simulink model "starshotsimv2"  (R2017a)
settings: Solver=VariableStepAuto  StartTime=0.0  StopTime=600  RelTol=1e-3
values from neighbouring files (symbols this model uses):
  B0 = 3.12e-5    (= 3.12e-05)    [starshot_DC_KD_setupv2.m]    (also in starshot_IC_initv2.m)
  G = 6.67e-11    [starshot_DC_KD_setupv2.m]    (also in starshot_IC_initv2.m)
  M_Earth = 5.972e24    (= 5.972e+24)    [starshot_DC_KD_setupv2.m]    (also in starshot_IC_initv2.m)
  mu_0 = 4*pi*(10^-7)    (= 1.25663706144e-06)    [starshot_DC_KD_setupv2.m]    (also in starshot_IC_initv2.m)
  n = 1000    [starshot_DC_KD_setupv2.m]    (also in starshot_IC_initv2.m = 500)
  omegacmd = [starshot.cmd.p,starshot.cmd.q,starshot.cmd.r]'    [starshot_IC_initv2.m]
  q0 = [qmatlab(2:4),qmatlab(1)]'    [starshot_DC_KD_setupv2.m]    (also in starshot_IC_initv2.m)
  R_Earth = 6.378e6    (= 6378000)    [starshot_DC_KD_setupv2.m]    (also in starshot_IC_initv2.m)
undefined symbols (not defined in the file or in its folder): qcmd, starshot
libraries: vrlib x2
settings Model: Creator=armen  LastModifiedBy=armen

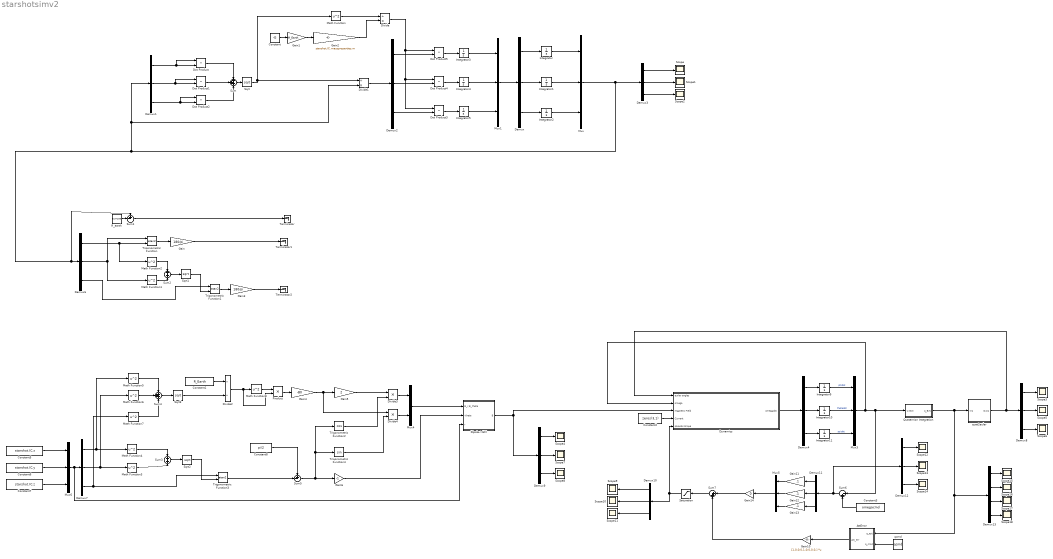
== system starshotsimv2 ==
  AttError : Subsystem
  Constant : Constant  Value=-G
  Constant1 : Constant  Value=R_Earth
  Constant2 : Constant  Value=zeros(3,1)
  Constant3 : Constant  Value=omegacmd
  Constant5 : Constant  Value=starshot.IC.x
  Constant6 : Constant  Value=starshot.IC.y
  Constant7 : Constant  Value=starshot.IC.z
  Constant8 : Constant  Value=pi/2
  Demux{,1..4,6..12} (12 alike) : Demux  Outputs=3
  Demux13 : Demux
  Dipole->ECI : Subsystem
  Divide : Product  Inputs=/*
  Divide1 : Product  Inputs=/*
  Divide2 : Product  Inputs=*/
  Divide3 : Product  Inputs=**
  Divide4 : Product  Inputs=**
  Dot Product{,1..5} (6 alike) : DotProduct  InputSameDT=on  OutDataTypeStr=Inherit: Inherit via internal rule
  Dynamics : Subsystem
  Gain : Gain  Gain=180/pi
  Gain1 : Gain  Gain=M_Earth
  Gain10 : Gain  Gain=[1,0,0;0,1,0;0,0,0,]  Multiplication=Matrix(K*u)
  Gain11 : Gain  Gain=.1
  Gain12 : Gain  Gain=.1
  Gain13 : Gain  Gain=.1
  Gain14 : Gain  Gain=0
  Gain2 : Gain  Gain=starshot.IC.massproperties.m
  Gain3 : Gain  Gain=180/pi
  Gain4 : Gain  Gain=-B0
  Gain5 : Gain  Gain=2
  Gain6 : Gain  Gain=-1
  Integrator : Integrator  InitialCondition=starshot.IC.x
  Integrator1 : Integrator  InitialCondition=starshot.IC.y
  Integrator10 : Integrator  InitialCondition=starshot.IC.thetadot
  Integrator11 : Integrator  InitialCondition=starshot.IC.psidot
  Integrator2 : Integrator  InitialCondition=starshot.IC.z
  Integrator3 : Integrator  InitialCondition=starshot.IC.xdot
  Integrator4 : Integrator  InitialCondition=starshot.IC.ydot
  Integrator5 : Integrator  InitialCondition=starshot.IC.zdot
  Integrator9 : Integrator  InitialCondition=starshot.IC.phidot
  Math Function{,1..8} (9 alike) : Math  Operator=square  SaturateOnIntegerOverflow=on
  Mux{,1,3,5..6} (5 alike) : Mux  Inputs=3
  Mux4 : Mux  Inputs=2
  Product : Product
  Quaternion Integration : Subsystem
  R_earth : Constant  Value=6.371e6
  Saturation : Saturate  UpperLimit=1e-4  LowerLimit=-1e-4
  Scope{,1..18} (19 alike) : Scope
  Sqrt{,1..3} (4 alike) : Sqrt  SaturateOnIntegerOverflow=on
  Sum : Sum  Inputs=+++
  Sum1 : Sum  Inputs=+-|
  Sum2 : Sum
  Sum3 : Sum
  Sum4 : Sum  Inputs=+++
  Sum5 : Sum  Inputs=+-|
  Sum6 : Sum  Inputs=|-+
  Sum7 : Sum  Inputs=|++
  Terminator : Terminator
  Terminator1 : Terminator
  Terminator2 : Terminator
  Trigonometric Function : Trigonometry  Operator=atan2
  Trigonometric Function1 : Trigonometry  Operator=atan2
  Trigonometric Function2 : Trigonometry  Operator=cos
  Trigonometric Function3 : Trigonometry  Operator=atan2
  Trigonometric Function4 : Trigonometry
  qcmd : Constant  Value=qcmd
  quat2euler : Subsystem
  wires:
  Integrator/1 -> Mux/1
  Integrator2/1 -> Mux/3
  Integrator1/1 -> Mux/2
  Demux/3 -> Integrator2/1
  Demux/2 -> Integrator1/1
  Demux/1 -> Integrator/1
  Mux1/1 -> Demux/1
  Integrator5/1 -> Mux1/3
  Integrator4/1 -> Mux1/2
  Integrator3/1 -> Mux1/1
  Demux1/1 -> Dot Product/1, Dot Product/2
  Demux1/2 -> Dot Product1/1, Dot Product1/2
  Demux1/3 -> Dot Product2/1, Dot Product2/2
  Dot Product1/1 -> Sum/2
  Dot Product2/1 -> Sum/3
  Dot Product/1 -> Sum/1
  Sum/1 -> Sqrt/1
  Constant/1 -> Gain1/1
  Sqrt/1 -> Math Function/1, Divide1/1
  Gain1/1 -> Gain2/1
  Gain2/1 -> Divide/2
  Math Function/1 -> Divide/1
  Divide/1 -> Dot Product3/1, Dot Product4/1, Dot Product5/1
  Demux2/3 -> Dot Product3/2
  Demux2/2 -> Dot Product4/2
  Demux2/1 -> Dot Product5/2
  Dot Product5/1 -> Integrator3/1
  Dot Product4/1 -> Integrator4/1
  Dot Product3/1 -> Integrator5/1
  Divide1/1 -> Demux2/1
  Demux3/1 -> Scope/1
  Demux3/2 -> Scope1/1
  Demux3/3 -> Scope2/1
  Integrator9/1 -> Mux3/1  "phidot"
  Integrator10/1 -> Mux3/2  "thetadot"
  Integrator11/1 -> Mux3/3  "psidot"
  Demux4/3 -> Integrator11/1
  Demux4/2 -> Integrator10/1
  Demux4/1 -> Integrator9/1
  Sum1/1 -> Terminator/1
  R_earth/1 -> Sum1/2
  Demux6/1 -> Math Function2/1, Trigonometric Function/2
  Demux6/2 -> Trigonometric Function/1, Math Function1/1
  Demux6/3 -> Trigonometric Function1/1
  Math Function2/1 -> Sum2/1
  Math Function1/1 -> Sum2/2
  Sum2/1 -> Sqrt1/1
  Sqrt1/1 -> Trigonometric Function1/2
  Trigonometric Function/1 -> Gain/1
  Trigonometric Function1/1 -> Gain3/1
  Gain/1 -> Terminator1/1
  Gain3/1 -> Terminator2/1
  Dynamics/1(omegadot) -> Demux4/1
  Sqrt2/1 -> Trigonometric Function3/2
  Sum3/1 -> Sqrt2/1
  Math Function3/1 -> Sum3/2
  Math Function4/1 -> Sum3/1
  Demux7/3 -> Math Function7/1, Trigonometric Function3/1
  Demux7/2 -> Math Function6/1, Math Function3/1
  Demux7/1 -> Math Function5/1, Math Function4/1
  Mux/1 -> Sum1/1, Demux6/1, Divide1/2, Demux1/1, Demux3/1
  Math Function6/1 -> Sum4/2
  Math Function5/1 -> Sum4/1
  Math Function7/1 -> Sum4/3
  Sum4/1 -> Sqrt3/1
  Sqrt3/1 -> Divide2/2
  Constant1/1 -> Divide2/1
  Divide2/1 -> Product/2, Math Function8/1
  Math Function8/1 -> Product/1
  Product/1 -> Gain4/1
  Gain4/1 -> Gain5/1, Divide4/1
  Gain5/1 -> Divide3/1
  Trigonometric Function2/1 -> Divide3/2
  Trigonometric Function4/1 -> Divide4/2
  Divide3/1 -> Mux4/1
  Divide4/1 -> Mux4/2
  Mux4/1 -> Dipole->ECI/1(B_r,B_theta)
  Gain6/1 -> Dipole->ECI/2(-theta)
  Demux9/3 -> Scope8/1
  Demux9/1 -> Scope4/1
  Demux9/2 -> Scope7/1
  Dipole->ECI/1(B) -> Demux9/1, Dynamics/3(Magnetic Field)
  Mux6/1 -> Dipole->ECI/3(r), Demux7/1
  Constant7/1 -> Mux6/3
  Constant6/1 -> Mux6/2
  Constant5/1 -> Mux6/1
  Demux8/2 -> Scope5/1
  Demux8/1 -> Scope3/1
  Demux8/3 -> Scope6/1
  Trigonometric Function3/1 -> Sum5/2
  Constant8/1 -> Sum5/1
  Sum5/1 -> Trigonometric Function2/1, Trigonometric Function4/1, Gain6/1
  quat2euler/1(Out1) -> Dynamics/1(eurler angles), Demux8/1
  AttError/1(att_err) -> Gain10/1
  qcmd/1 -> AttError/2(q_cmd)
  Constant2/1 -> Dynamics/4("Current ")
  Gain10/1 -> Sum7/2
  Demux10/1 -> Scope9/1
  Demux10/2 -> Scope10/1
  Demux10/3 -> Scope11/1
  Demux11/3 -> Gain13/1
  Gain13/1 -> Mux5/3
  Demux11/2 -> Gain12/1
  Gain12/1 -> Mux5/2
  Demux11/1 -> Gain11/1
  Gain11/1 -> Mux5/1
  Mux5/1 -> Gain14/1
  Sum6/1 -> Demux12/1, Demux11/1
  Constant3/1 -> Sum6/2
  Gain14/1 -> Sum7/1
  Sum7/1 -> Saturation/1
  Saturation/1 -> Demux10/1, Dynamics/5(pseudo-torque)
  Mux3/1 -> Dynamics/2(omega), Sum6/1, Quaternion Integration/1(w B/N)
  Demux12/3 -> Scope14/1
  Demux12/1 -> Scope12/1
  Demux12/2 -> Scope13/1
  Quaternion Integration/1(q_B/N) -> AttError/1(q_est), Demux13/1, quat2euler/1(In1)
  Demux13/1 -> Scope15/1
  Demux13/2 -> Scope16/1
  Demux13/3 -> Scope17/1
  Demux13/4 -> Scope18/1

== system starshotsimv2/AttError ==
  q_est : Inport  PortDimensions=4
  q_cmd : Inport  Port=2  PortDimensions=4
  Demux : Demux
  Gain : Gain  Gain=2  SaturateOnIntegerOverflow=on  OutDataTypeStr=Inherit: Same as input  ParamDataTypeStr=Inherit: Same as input
  Mux : Mux  Inputs=3
  Terminator : Terminator
  qconjMult : Subsystem
  att_err : Outport
  wires:
  Demux/4 -> Terminator/1
  Gain/1 -> att_err/1
  Mux/1 -> Gain/1
  Demux/3 -> Mux/3
  Demux/2 -> Mux/2
  Demux/1 -> Mux/1
  qconjMult/1(q_err) -> Demux/1
  q_est/1 -> qconjMult/2(q_est)
  q_cmd/1 -> qconjMult/1(q_cmd)

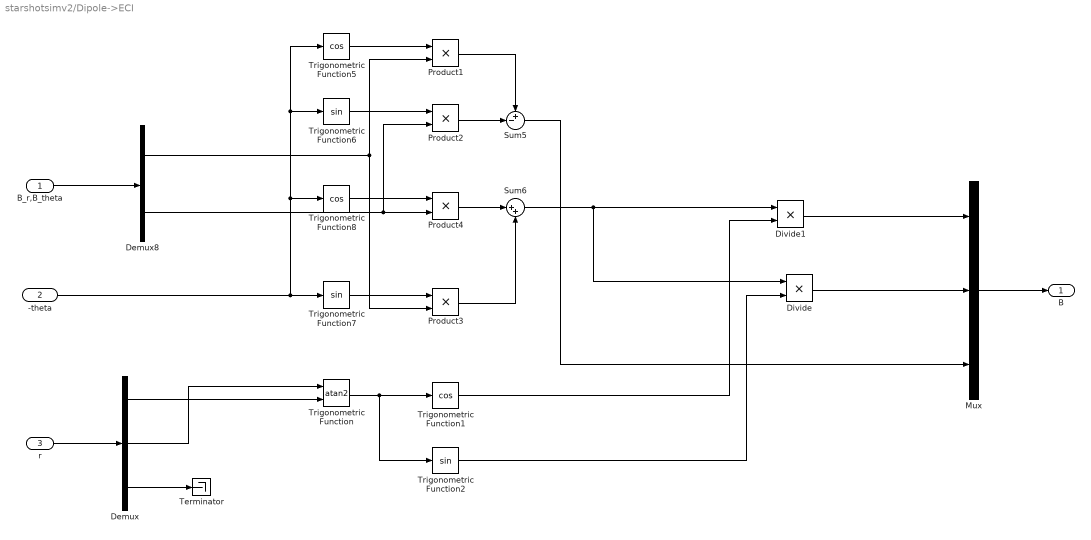
== system starshotsimv2/Dipole->ECI ==
  B_r,B_theta : Inport
  -theta : Inport  Port=2
  r : Inport  Port=3
  Demux : Demux  Outputs=3
  Demux8 : Demux  Outputs=2
  Divide : Product  Inputs=**
  Divide1 : Product  Inputs=**
  Mux : Mux  Inputs=3
  Product{1..4} (4 alike) : Product
  Sum5 : Sum  Inputs=+-|
  Sum6 : Sum  Inputs=|++
  Terminator : Terminator
  Trigonometric Function : Trigonometry  Operator=atan2
  Trigonometric Function1 : Trigonometry  Operator=cos
  Trigonometric Function2 : Trigonometry
  Trigonometric Function5 : Trigonometry  Operator=cos
  Trigonometric Function6 : Trigonometry
  Trigonometric Function7 : Trigonometry
  Trigonometric Function8 : Trigonometry  Operator=cos
  B : Outport
  wires:
  -theta/1 -> Trigonometric Function5/1, Trigonometric Function6/1, Trigonometric Function8/1, Trigonometric Function7/1
  Product4/1 -> Sum6/1
  Product3/1 -> Sum6/2
  Demux8/1 -> Product3/2, Product1/2
  Demux8/2 -> Product2/2, Product4/2
  Trigonometric Function5/1 -> Product1/1
  Product2/1 -> Sum5/2
  Trigonometric Function7/1 -> Product3/1
  B_r,B_theta/1 -> Demux8/1
  Sum5/1 -> Mux/3
  Trigonometric Function8/1 -> Product4/1
  Trigonometric Function6/1 -> Product2/1
  Sum6/1 -> Divide1/1, Divide/1
  Product1/1 -> Sum5/1
  r/1 -> Demux/1
  Demux/3 -> Terminator/1
  Demux/2 -> Trigonometric Function/1
  Demux/1 -> Trigonometric Function/2
  Trigonometric Function/1 -> Trigonometric Function1/1, Trigonometric Function2/1
  Trigonometric Function1/1 -> Divide1/2
  Trigonometric Function2/1 -> Divide/2
  Mux/1 -> B/1
  Divide1/1 -> Mux/1
  Divide/1 -> Mux/2

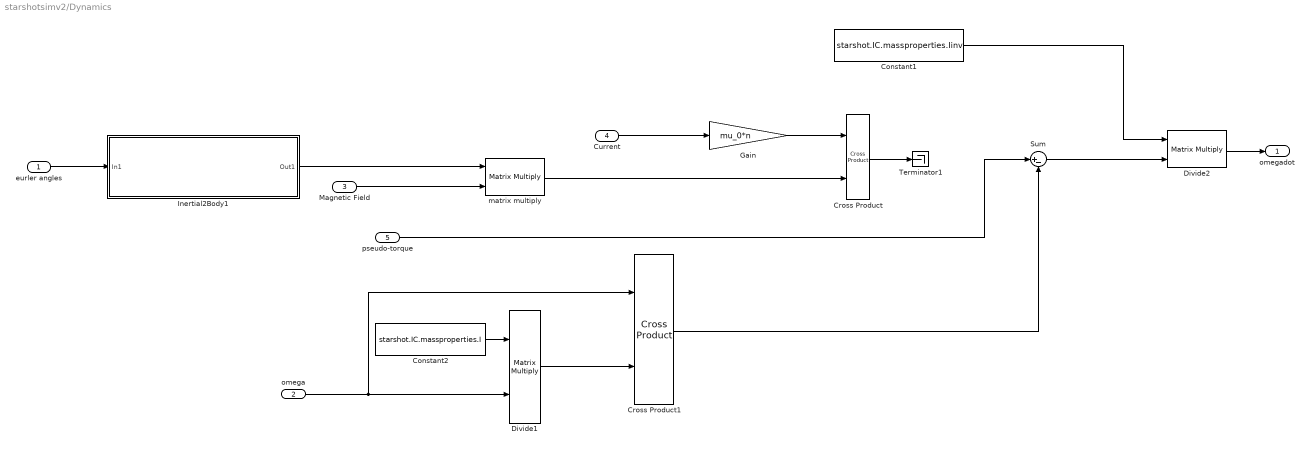
== system starshotsimv2/Dynamics ==
  eurler angles : Inport
  omega : Inport  Port=2
  Magnetic Field : Inport  Port=3
  "Current " : Inport  Port=4
  pseudo-torque : Inport  Port=5
  Constant1 : Constant  Value=starshot.IC.massproperties.Iinv  VectorParams1D=off
  Constant2 : Constant  Value=starshot.IC.massproperties.I  VectorParams1D=off
  Cross Product : vrlib/Utilities/Cross Product
      settings: SourceProductBaseCode=VR
  Cross Product1 : vrlib/Utilities/Cross Product
      settings: SourceProductBaseCode=VR
  Divide1 : Product  Inputs=**  Multiplication=Matrix(*)
  Divide2 : Product  Inputs=**  Multiplication=Matrix(*)
  Gain : Gain  Gain=mu_0*n
  Inertial2Body1 : Subsystem
  Sum : Sum  Inputs=|+-
  Terminator1 : Terminator
  "matrix multiply " : Product  Inputs=**  Multiplication=Matrix(*)
  omegadot : Outport
  wires:
  eurler angles/1 -> Inertial2Body1/1(In1)
  Inertial2Body1/1(Out1) -> "matrix multiply "/1
  omega/1 -> Divide1/2, Cross Product1/1
  Constant2/1 -> Divide1/1
  Magnetic Field/1 -> "matrix multiply "/2
  "Current "/1 -> Gain/1
  "matrix multiply "/1 -> Cross Product/2
  Gain/1 -> Cross Product/1
  Cross Product/1 -> Terminator1/1
  Divide1/1 -> Cross Product1/2
  Cross Product1/1 -> Sum/2
  Sum/1 -> Divide2/2
  Constant1/1 -> Divide2/1
  Divide2/1 -> omegadot/1
  pseudo-torque/1 -> Sum/1

== system starshotsimv2/Quaternion Integration ==
  w B/N : Inport
  Integrator1 : Integrator  InitialCondition=q0
  q_normalize : Subsystem
  qderiv : Subsystem
  q_B/N : Outport
  wires:
  w B/N/1 -> qderiv/1(w)
  q_normalize/1(q_out) -> qderiv/2(q), q_B/N/1
  Integrator1/1 -> q_normalize/1(q_in)
  qderiv/1(qd) -> Integrator1/1

== system starshotsimv2/quat2euler ==
  In1 : Inport
  Mux : Mux  Inputs=3
  Subsystem : Subsystem
  Subsystem1 : Subsystem
  q2phi : Subsystem
  Out1 : Outport
  wires:
  In1/1 -> Subsystem/1(q), Subsystem1/1(q), q2phi/1(q)
  Mux/1 -> Out1/1
  q2phi/1(phi) -> Mux/1
  Subsystem1/1(theta) -> Mux/2
  Subsystem/1(psi) -> Mux/3

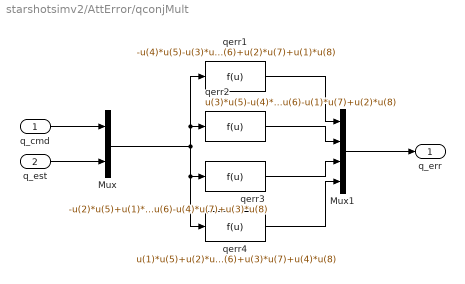
== system starshotsimv2/AttError/qconjMult ==
  q_cmd : Inport
  q_est : Inport  Port=2
  Mux : Mux  Inputs=2
  Mux1 : Mux
  qerr1 : Fcn  Expr=-u(4)*u(5)-u(3)*u(6)+u(2)*u(7)+u(1)*u(8)
  qerr2 : Fcn  Expr=u(3)*u(5)-u(4)*u(6)-u(1)*u(7)+u(2)*u(8)
  qerr3 : Fcn  Expr=-u(2)*u(5)+u(1)*u(6)-u(4)*u(7)+u(3)*u(8)
  qerr4 : Fcn  Expr=u(1)*u(5)+u(2)*u(6)+u(3)*u(7)+u(4)*u(8)
  q_err : Outport
  wires:
  Mux1/1 -> q_err/1
  qerr4/1 -> Mux1/4
  qerr3/1 -> Mux1/3
  qerr2/1 -> Mux1/2
  qerr1/1 -> Mux1/1
  Mux/1 -> qerr4/1, qerr3/1, qerr2/1, qerr1/1
  q_est/1 -> Mux/2
  q_cmd/1 -> Mux/1

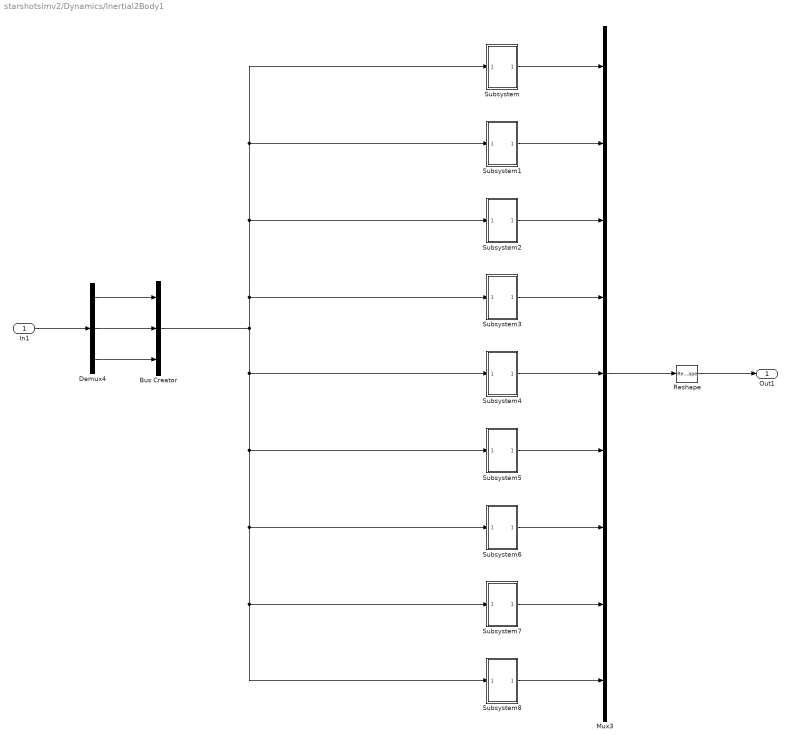
== system starshotsimv2/Dynamics/Inertial2Body1 ==
  In1 : Inport
  Bus Creator : BusCreator  Inputs=3
  Demux4 : Demux  Outputs=3
  Mux3 : Mux  Inputs=9
  Reshape : Reshape  OutputDimensionality=Customize  OutputDimensions=[3,3]
  Subsystem : Subsystem
  Subsystem1 : Subsystem
  Subsystem2 : Subsystem
  Subsystem3 : Subsystem
  Subsystem4 : Subsystem
  Subsystem5 : Subsystem
  Subsystem6 : Subsystem
  Subsystem7 : Subsystem
  Subsystem8 : Subsystem
  Out1 : Outport
  wires:
  Reshape/1 -> Out1/1
  Subsystem3/1(Out1) -> Mux3/4
  Subsystem4/1(Out1) -> Mux3/5
  Subsystem6/1(Out1) -> Mux3/7
  Subsystem2/1(Out1) -> Mux3/3
  Subsystem8/1(Out1) -> Mux3/9
  Subsystem7/1(Out1) -> Mux3/8
  Subsystem5/1(Out1) -> Mux3/6
  Subsystem1/1(Out1) -> Mux3/2
  Subsystem/1(Out1) -> Mux3/1
  Bus Creator/1 -> Subsystem4/1(In1), Subsystem5/1(In1), Subsystem8/1(In1), Subsystem7/1(In1), Subsystem6/1(In1), Subsystem3/1(In1), Subsystem1/1(In1), Subsystem/1(In1), Subsystem2/1(In1)
  Demux4/3 -> Bus Creator/3
  In1/1 -> Demux4/1
  Demux4/1 -> Bus Creator/1
  Demux4/2 -> Bus Creator/2
  Mux3/1 -> Reshape/1

== system starshotsimv2/Quaternion Integration/q_normalize ==
  q_in : Inport  PortDimensions=4
  Dot Product : DotProduct  InputSameDT=on  OutDataTypeStr=Inherit: Inherit via internal rule
  Math Function : Math  Operator=sqrt  SaturateOnIntegerOverflow=on
  Product : Product  Inputs=*/  SaturateOnIntegerOverflow=on  InputSameDT=on  OutDataTypeStr=Inherit: Same as first input
  q_out : Outport
  wires:
  Product/1 -> q_out/1
  Math Function/1 -> Product/2
  Dot Product/1 -> Math Function/1
  q_in/1 -> Dot Product/2, Dot Product/1, Product/1

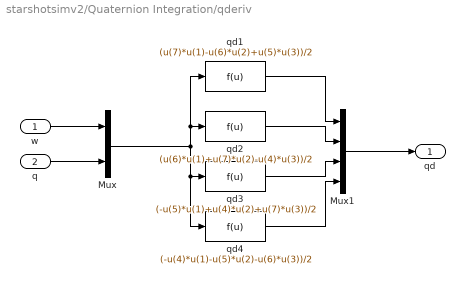
== system starshotsimv2/Quaternion Integration/qderiv ==
  w : Inport
  q : Inport  Port=2
  Mux : Mux  Inputs=2
  Mux1 : Mux
  qd1 : Fcn  Expr=(u(7)*u(1)-u(6)*u(2)+u(5)*u(3))/2
  qd2 : Fcn  Expr=(u(6)*u(1)+u(7)*u(2)-u(4)*u(3))/2
  qd3 : Fcn  Expr=(-u(5)*u(1)+u(4)*u(2)+u(7)*u(3))/2
  qd4 : Fcn  Expr=(-u(4)*u(1)-u(5)*u(2)-u(6)*u(3))/2
  qd : Outport
  wires:
  Mux1/1 -> qd/1
  qd4/1 -> Mux1/4
  qd3/1 -> Mux1/3
  qd2/1 -> Mux1/2
  qd1/1 -> Mux1/1
  Mux/1 -> qd4/1, qd3/1, qd2/1, qd1/1
  q/1 -> Mux/2
  w/1 -> Mux/1

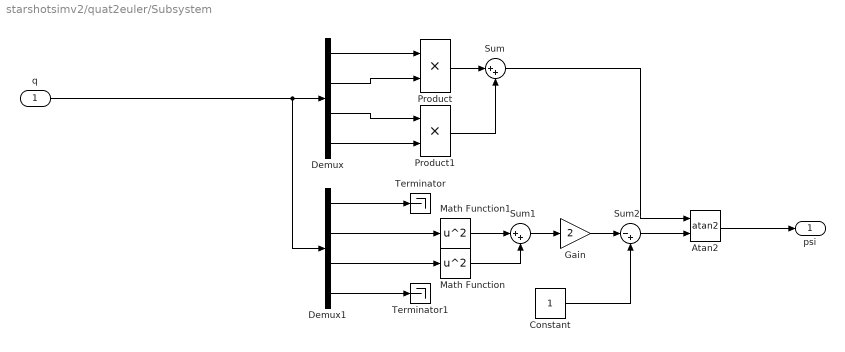
== system starshotsimv2/quat2euler/Subsystem ==
  q : Inport
  Atan2 : Trigonometry  Operator=atan2
  Constant : Constant
  Demux : Demux
  Demux1 : Demux
  Gain : Gain  Gain=2
  Math Function : Math  Operator=square  SaturateOnIntegerOverflow=on
  Math Function1 : Math  Operator=square  SaturateOnIntegerOverflow=on
  Product : Product
  Product1 : Product
  Sum : Sum  Inputs=|++
  Sum1 : Sum  Inputs=|++
  Sum2 : Sum  Inputs=|-+
  Terminator : Terminator
  Terminator1 : Terminator
  psi : Outport
  wires:
  Sum2/1 -> Atan2/2
  Math Function1/1 -> Sum1/1
  Demux/2 -> Product/2
  Demux/3 -> Product1/1
  Demux/4 -> Product1/2
  Product1/1 -> Sum/2
  Product/1 -> Sum/1
  Sum1/1 -> Gain/1
  Atan2/1 -> psi/1
  Sum/1 -> Atan2/1
  Demux1/2 -> Math Function1/1
  Demux1/4 -> Terminator1/1
  q/1 -> Demux1/1, Demux/1
  Demux1/3 -> Math Function/1
  Gain/1 -> Sum2/1
  Demux/1 -> Product/1
  Demux1/1 -> Terminator/1
  Constant/1 -> Sum2/2
  Math Function/1 -> Sum1/2

== system starshotsimv2/quat2euler/Subsystem1 ==
  q : Inport
  Demux : Demux
  Gain : Gain  Gain=2
  Product : Product
  Product1 : Product
  Sum : Sum  Inputs=-+|
  Trigonometric Function : Trigonometry  Operator=asin
  theta : Outport
  wires:
  Sum/1 -> Gain/1
  Trigonometric Function/1 -> theta/1
  Demux/2 -> Product/1
  Product1/1 -> Sum/1
  Gain/1 -> Trigonometric Function/1
  Demux/1 -> Product1/1
  Demux/4 -> Product/2
  Demux/3 -> Product1/2
  Product/1 -> Sum/2
  q/1 -> Demux/1

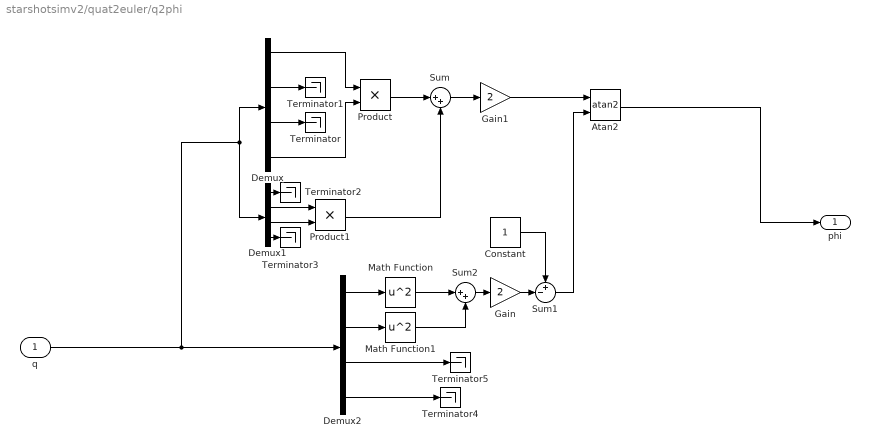
== system starshotsimv2/quat2euler/q2phi ==
  q : Inport
  Atan2 : Trigonometry  Operator=atan2
  Constant : Constant
  Demux : Demux
  Demux1 : Demux
  Demux2 : Demux
  Gain : Gain  Gain=2
  Gain1 : Gain  Gain=2
  Math Function : Math  Operator=square  SaturateOnIntegerOverflow=on
  Math Function1 : Math  Operator=square  SaturateOnIntegerOverflow=on
  Product : Product
  Product1 : Product
  Sum : Sum  Inputs=|++
  Sum1 : Sum  Inputs=+-|
  Sum2 : Sum  Inputs=|++
  Terminator{,1..5} (6 alike) : Terminator
  phi : Outport
  wires:
  Demux2/4 -> Terminator4/1
  Demux1/2 -> Product1/1
  Product/1 -> Sum/1
  Demux2/1 -> Math Function/1
  Atan2/1 -> phi/1
  Sum/1 -> Gain1/1
  Demux/3 -> Terminator/1
  Demux1/4 -> Terminator3/1
  Demux2/3 -> Terminator5/1
  Product1/1 -> Sum/2
  Demux/2 -> Terminator1/1
  Demux1/1 -> Terminator2/1
  Demux/4 -> Product/2
  Demux1/3 -> Product1/2
  Demux/1 -> Product/1
  Math Function1/1 -> Sum2/2
  Sum2/1 -> Gain/1
  Demux2/2 -> Math Function1/1
  Gain/1 -> Sum1/2
  Constant/1 -> Sum1/1
  Gain1/1 -> Atan2/1
  Sum1/1 -> Atan2/2
  q/1 -> Demux1/1, Demux/1, Demux2/1
  Math Function/1 -> Sum2/1

== system starshotsimv2/Dynamics/Inertial2Body1/Subsystem ==
  In1 : Inport
  Bus Selector : BusSelector  OutputSignals=signal1,signal3
  Product4 : Product
  Trigonometric Function : Trigonometry  Operator=cos
  Trigonometric Function1 : Trigonometry  Operator=cos
  Out1 : Outport
  wires:
  In1/1 -> Bus Selector/1
  Product4/1 -> Out1/1
  Trigonometric Function/1 -> Product4/1
  Trigonometric Function1/1 -> Product4/2
  Bus Selector/1 -> Trigonometric Function/1  "<signal1>"
  Bus Selector/2 -> Trigonometric Function1/1  "<signal3>"

== system starshotsimv2/Dynamics/Inertial2Body1/Subsystem1 ==
  In1 : Inport
  Bus Selector1 : BusSelector  OutputSignals=signal1,signal3
  Product5 : Product
  Trigonometric Function2 : Trigonometry  Operator=cos
  Trigonometric Function3 : Trigonometry
  Out1 : Outport
  wires:
  In1/1 -> Bus Selector1/1
  Product5/1 -> Out1/1
  Trigonometric Function2/1 -> Product5/1
  Bus Selector1/1 -> Trigonometric Function2/1  "<signal1>"
  Trigonometric Function3/1 -> Product5/2
  Bus Selector1/2 -> Trigonometric Function3/1  "<signal3>"

== system starshotsimv2/Dynamics/Inertial2Body1/Subsystem2 ==
  In1 : Inport
  Bus Selector2 : BusSelector  OutputSignals=signal3
  Gain : Gain  Gain=-1
  Trigonometric Function4 : Trigonometry
  Out1 : Outport
  wires:
  Gain/1 -> Out1/1
  In1/1 -> Bus Selector2/1
  Bus Selector2/1 -> Trigonometric Function4/1  "<signal3>"
  Trigonometric Function4/1 -> Gain/1

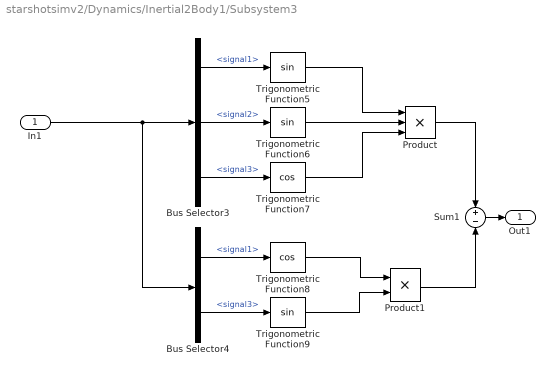
== system starshotsimv2/Dynamics/Inertial2Body1/Subsystem3 ==
  In1 : Inport
  Bus Selector3 : BusSelector  OutputSignals=signal1,signal2,signal3
  Bus Selector4 : BusSelector  OutputSignals=signal1,signal3
  Product : Product  Inputs=3
  Product1 : Product
  Sum1 : Sum  Inputs=+-
  Trigonometric Function5 : Trigonometry
  Trigonometric Function6 : Trigonometry
  Trigonometric Function7 : Trigonometry  Operator=cos
  Trigonometric Function8 : Trigonometry  Operator=cos
  Trigonometric Function9 : Trigonometry
  Out1 : Outport
  wires:
  Sum1/1 -> Out1/1
  In1/1 -> Bus Selector3/1, Bus Selector4/1
  Trigonometric Function7/1 -> Product/3
  Trigonometric Function9/1 -> Product1/2
  Product/1 -> Sum1/1
  Product1/1 -> Sum1/2
  Trigonometric Function5/1 -> Product/1
  Trigonometric Function6/1 -> Product/2
  Bus Selector4/1 -> Trigonometric Function8/1  "<signal1>"
  Bus Selector3/3 -> Trigonometric Function7/1  "<signal3>"
  Bus Selector3/1 -> Trigonometric Function5/1  "<signal1>"
  Bus Selector4/2 -> Trigonometric Function9/1  "<signal3>"
  Trigonometric Function8/1 -> Product1/1
  Bus Selector3/2 -> Trigonometric Function6/1  "<signal2>"

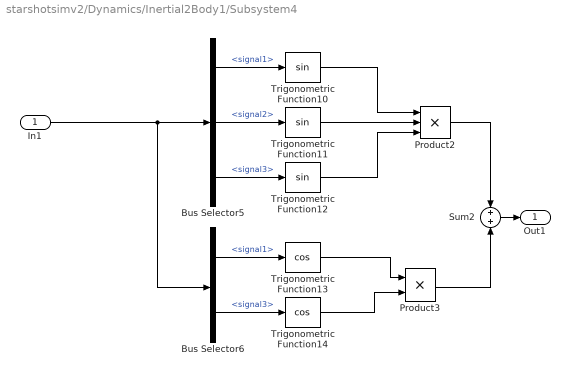
== system starshotsimv2/Dynamics/Inertial2Body1/Subsystem4 ==
  In1 : Inport
  Bus Selector5 : BusSelector  OutputSignals=signal1,signal2,signal3
  Bus Selector6 : BusSelector  OutputSignals=signal1,signal3
  Product2 : Product  Inputs=3
  Product3 : Product
  Sum2 : Sum
  Trigonometric Function10 : Trigonometry
  Trigonometric Function11 : Trigonometry
  Trigonometric Function12 : Trigonometry
  Trigonometric Function13 : Trigonometry  Operator=cos
  Trigonometric Function14 : Trigonometry  Operator=cos
  Out1 : Outport
  wires:
  Sum2/1 -> Out1/1
  In1/1 -> Bus Selector6/1, Bus Selector5/1
  Trigonometric Function12/1 -> Product2/3
  Bus Selector6/1 -> Trigonometric Function13/1  "<signal1>"
  Bus Selector5/1 -> Trigonometric Function10/1  "<signal1>"
  Bus Selector5/3 -> Trigonometric Function12/1  "<signal3>"
  Trigonometric Function10/1 -> Product2/1
  Bus Selector6/2 -> Trigonometric Function14/1  "<signal3>"
  Trigonometric Function11/1 -> Product2/2
  Bus Selector5/2 -> Trigonometric Function11/1  "<signal2>"
  Trigonometric Function13/1 -> Product3/1
  Trigonometric Function14/1 -> Product3/2
  Product2/1 -> Sum2/1
  Product3/1 -> Sum2/2

== system starshotsimv2/Dynamics/Inertial2Body1/Subsystem5 ==
  In1 : Inport
  Bus Selector7 : BusSelector  OutputSignals=signal1,signal2
  Product6 : Product
  Trigonometric Function15 : Trigonometry
  Trigonometric Function16 : Trigonometry  Operator=cos
  Out1 : Outport
  wires:
  In1/1 -> Bus Selector7/1
  Product6/1 -> Out1/1
  Trigonometric Function15/1 -> Product6/1
  Trigonometric Function16/1 -> Product6/2
  Bus Selector7/1 -> Trigonometric Function15/1  "<signal1>"
  Bus Selector7/2 -> Trigonometric Function16/1  "<signal2>"

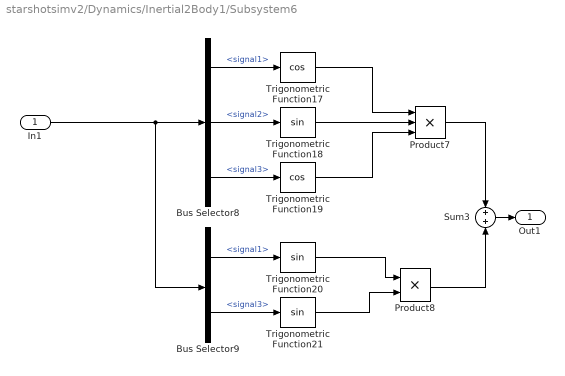
== system starshotsimv2/Dynamics/Inertial2Body1/Subsystem6 ==
  In1 : Inport
  Bus Selector8 : BusSelector  OutputSignals=signal1,signal2,signal3
  Bus Selector9 : BusSelector  OutputSignals=signal1,signal3
  Product7 : Product  Inputs=3
  Product8 : Product
  Sum3 : Sum
  Trigonometric Function17 : Trigonometry  Operator=cos
  Trigonometric Function18 : Trigonometry
  Trigonometric Function19 : Trigonometry  Operator=cos
  Trigonometric Function20 : Trigonometry
  Trigonometric Function21 : Trigonometry
  Out1 : Outport
  wires:
  In1/1 -> Bus Selector9/1, Bus Selector8/1
  Sum3/1 -> Out1/1
  Bus Selector8/1 -> Trigonometric Function17/1  "<signal1>"
  Bus Selector8/2 -> Trigonometric Function18/1  "<signal2>"
  Trigonometric Function18/1 -> Product7/2
  Trigonometric Function17/1 -> Product7/1
  Bus Selector8/3 -> Trigonometric Function19/1  "<signal3>"
  Trigonometric Function20/1 -> Product8/1
  Bus Selector9/1 -> Trigonometric Function20/1  "<signal1>"
  Trigonometric Function19/1 -> Product7/3
  Product7/1 -> Sum3/1
  Trigonometric Function21/1 -> Product8/2
  Bus Selector9/2 -> Trigonometric Function21/1  "<signal3>"
  Product8/1 -> Sum3/2

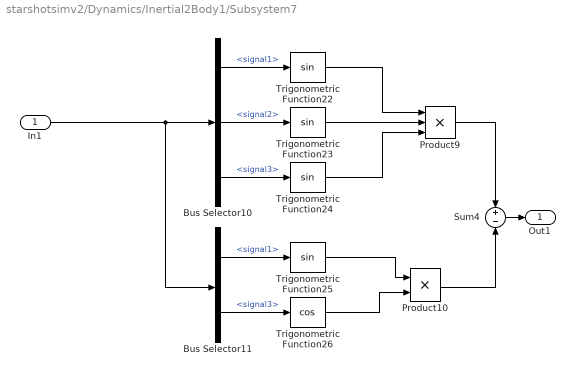
== system starshotsimv2/Dynamics/Inertial2Body1/Subsystem7 ==
  In1 : Inport
  Bus Selector10 : BusSelector  OutputSignals=signal1,signal2,signal3
  Bus Selector11 : BusSelector  OutputSignals=signal1,signal3
  Product10 : Product
  Product9 : Product  Inputs=3
  Sum4 : Sum  Inputs=+-
  Trigonometric Function{22..25} (4 alike) : Trigonometry
  Trigonometric Function26 : Trigonometry  Operator=cos
  Out1 : Outport
  wires:
  In1/1 -> Bus Selector10/1, Bus Selector11/1
  Sum4/1 -> Out1/1
  Product10/1 -> Sum4/2
  Product9/1 -> Sum4/1
  Trigonometric Function25/1 -> Product10/1
  Trigonometric Function26/1 -> Product10/2
  Trigonometric Function22/1 -> Product9/1
  Trigonometric Function23/1 -> Product9/2
  Trigonometric Function24/1 -> Product9/3
  Bus Selector11/2 -> Trigonometric Function26/1  "<signal3>"
  Bus Selector11/1 -> Trigonometric Function25/1  "<signal1>"
  Bus Selector10/3 -> Trigonometric Function24/1  "<signal3>"
  Bus Selector10/2 -> Trigonometric Function23/1  "<signal2>"
  Bus Selector10/1 -> Trigonometric Function22/1  "<signal1>"

== system starshotsimv2/Dynamics/Inertial2Body1/Subsystem8 ==
  In1 : Inport
  Bus Selector12 : BusSelector  OutputSignals=signal1,signal2
  Product11 : Product
  Trigonometric Function27 : Trigonometry  Operator=cos
  Trigonometric Function28 : Trigonometry  Operator=cos
  Out1 : Outport
  wires:
  Product11/1 -> Out1/1
  In1/1 -> Bus Selector12/1
  Bus Selector12/1 -> Trigonometric Function27/1  "<signal1>"
  Bus Selector12/2 -> Trigonometric Function28/1  "<signal2>"
  Trigonometric Function27/1 -> Product11/1
  Trigonometric Function28/1 -> Product11/2
